simulink model "Sim1"  (R2024b)
settings: Solver=VariableStepAuto  StartTime=0.0  StopTime=50  RelTol=1e-3
undefined symbols (not defined in the file or in its folder): eng, gbx, road, tire, veh
settings Model: Creator=amira  LastModifiedBy=Ali
settings OptimizationCC: ReuseModelBlockBuffer=off
settings RTWCC: GPUComputeCapability=3.5

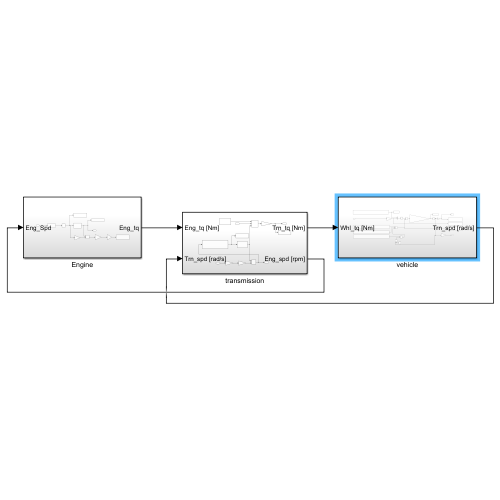
[thumbnail: Simulink's stored preview of the top-level diagram]
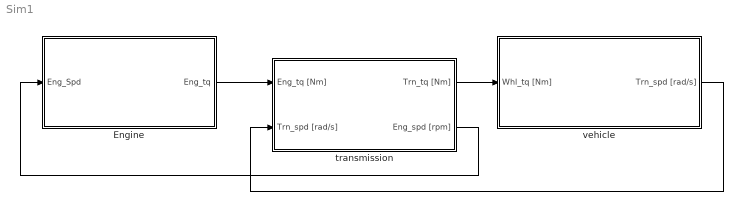
== system Sim1 ==
  Engine : Subsystem
  transmission : Subsystem
  vehicle : Subsystem
  wires:
  Engine/1(Eng_tq) -> transmission/1(Eng_tq [Nm])
  transmission/2(Eng_spd [rpm]) -> Engine/1(Eng_Spd)
  transmission/1(Trn_tq [Nm]) -> vehicle/1(Whl_tq [Nm])
  vehicle/1(Trn_spd [rad/s]) -> transmission/2(Trn_spd [rad/s])

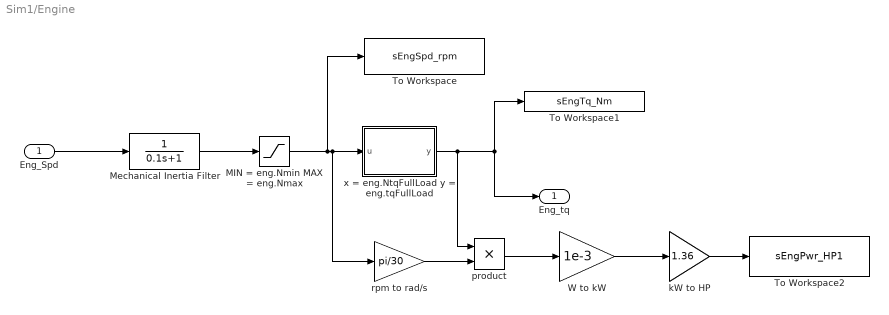
== system Sim1/Engine ==
  Eng_Spd : Inport
  MIN = eng.Nmin MAX = eng.Nmax : Saturate  UpperLimit=6500  LowerLimit=1000
  Mechanical Inertia Filter : TransferFcn  Denominator=[0.1 1]
  To Workspace : ToWorkspace  VariableName=sEngSpd_rpm  SaveFormat=Timeseries  SampleTime=-1
  To Workspace1 : ToWorkspace  VariableName=sEngTq_Nm  SaveFormat=Timeseries  SampleTime=-1
  To Workspace2 : ToWorkspace  VariableName=sEngPwr_HP1  SaveFormat=Timeseries  SampleTime=-1
  W to kW : Gain  Gain=1e-3
  kW to HP : Gain  Gain=1.36
  product : Product
  rpm to rad/s : Gain  Gain=pi/30
  x = eng.NtqFullLoad y = eng.tqFullLoad : MATLAB Function  TreatAsAtomicUnit=on
  Eng_tq : Outport
  wires:
  Eng_Spd/1 -> Mechanical Inertia Filter/1
  Mechanical Inertia Filter/1 -> MIN = eng.Nmin MAX = eng.Nmax/1
  MIN = eng.Nmin MAX = eng.Nmax/1 -> x = eng.NtqFullLoad y = eng.tqFullLoad/1(u), rpm to rad/s/1, To Workspace/1
  x = eng.NtqFullLoad y = eng.tqFullLoad/1(y) -> Eng_tq/1, To Workspace1/1, product/1
  rpm to rad/s/1 -> product/2
  product/1 -> W to kW/1
  W to kW/1 -> kW to HP/1
  kW to HP/1 -> To Workspace2/1

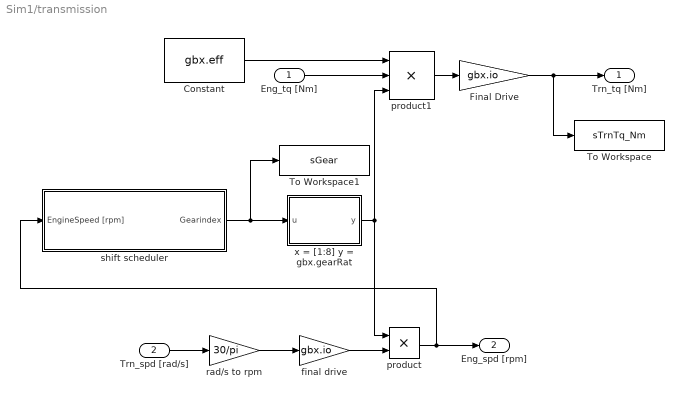
== system Sim1/transmission ==
  Eng_tq [Nm] : Inport
  Trn_spd [rad/s] : Inport  Port=2
  Constant : Constant  Value=gbx.eff
  Final Drive : Gain  Gain=gbx.io
  To Workspace : ToWorkspace  VariableName=sTrnTq_Nm  SaveFormat=Timeseries  SampleTime=-1
  To Workspace1 : ToWorkspace  VariableName=sGear  SaveFormat=Timeseries  SampleTime=-1
  final drive : Gain  Gain=gbx.io
  product : Product
  product1 : Product  Inputs=3
  rad/s to rpm : Gain  Gain=30/pi
  shift scheduler : Subsystem
  x = [1:8] y = gbx.gearRat : MATLAB Function  TreatAsAtomicUnit=on
  Trn_tq [Nm] : Outport
  Eng_spd [rpm] : Outport  Port=2
  wires:
  rad/s to rpm/1 -> final drive/1
  final drive/1 -> product/2
  x = [1:8] y = gbx.gearRat/1(y) -> product/1, product1/3
  Constant/1 -> product1/1
  Eng_tq [Nm]/1 -> product1/2
  product1/1 -> Final Drive/1
  Final Drive/1 -> Trn_tq [Nm]/1, To Workspace/1
  product/1 -> Eng_spd [rpm]/1, shift scheduler/1(EngineSpeed [rpm])
  shift scheduler/1(Gearindex) -> To Workspace1/1, x = [1:8] y = gbx.gearRat/1(u)
  Trn_spd [rad/s]/1 -> rad/s to rpm/1

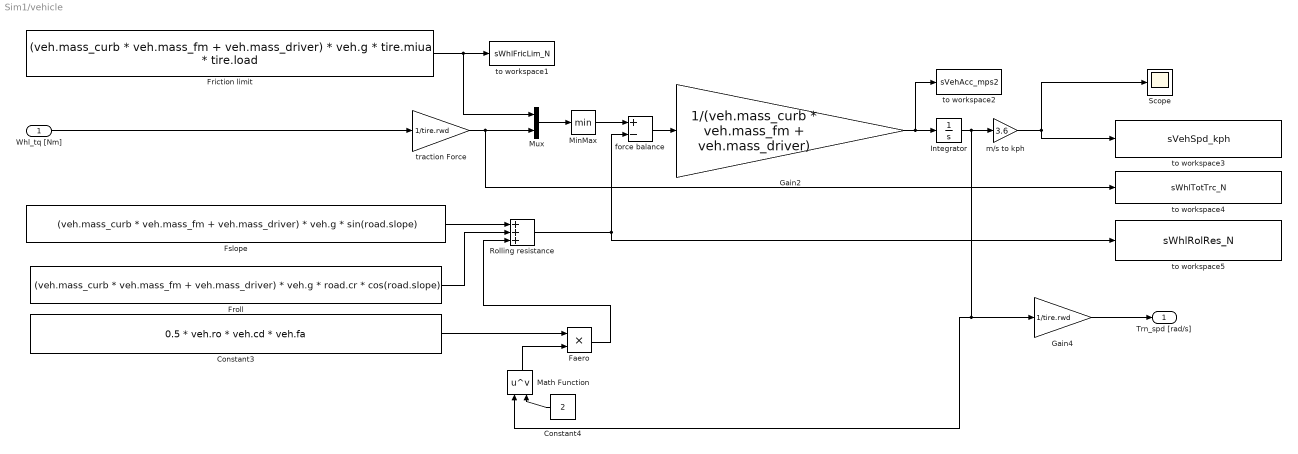
== system Sim1/vehicle ==
  Whl_tq [Nm] : Inport
  Constant3 : Constant  Value=0.5 * veh.ro * veh.cd * veh.fa
  Constant4 : Constant  Value=2
  Faero : Product
  Friction limit : Constant  Value=(veh.mass_curb * veh.mass_fm + veh.mass_driver) * veh.g * tire.miua * tire.load
  Froll : Constant  Value=(veh.mass_curb * veh.mass_fm + veh.mass_driver) * veh.g * road.cr * cos(road.slope)
  Fslope : Constant  Value=(veh.mass_curb * veh.mass_fm + veh.mass_driver) * veh.g * sin(road.slope)
  Gain2 : Gain  Gain=1/(veh.mass_curb * veh.mass_fm + veh.mass_driver)
  Gain4 : Gain  Gain=1/tire.rwd
  Integrator : Integrator
  Math Function : Math  Operator=pow  SignedPower=on
  MinMax : MinMax
  Mux : Mux  Inputs=2
  Rolling resistance : Sum  Inputs=+++
  Scope : Scope
  force balance : Sum  Inputs=+-
  m/s to kph : Gain  Gain=3.6
  to workspace1 : ToWorkspace  VariableName=sWhlFricLim_N  SaveFormat=Timeseries  SampleTime=-1
  to workspace2 : ToWorkspace  VariableName=sVehAcc_mps2  SaveFormat=Timeseries  SampleTime=-1
  to workspace3 : ToWorkspace  VariableName=sVehSpd_kph  SaveFormat=Timeseries  SampleTime=-1
  to workspace4 : ToWorkspace  VariableName=sWhlTotTrc_N  SaveFormat=Timeseries  SampleTime=-1
  to workspace5 : ToWorkspace  VariableName=sWhlRolRes_N  SaveFormat=Timeseries  SampleTime=-1
  traction Force : Gain  Gain=1/tire.rwd
  Trn_spd [rad/s] : Outport
  wires:
  Integrator/1 -> Math Function/1, Gain4/1, m/s to kph/1
  Whl_tq [Nm]/1 -> traction Force/1
  MinMax/1 -> force balance/1
  Gain4/1 -> Trn_spd [rad/s]/1
  Rolling resistance/1 -> force balance/2, to workspace5/1
  Fslope/1 -> Rolling resistance/1
  traction Force/1 -> to workspace4/1, Mux/2
  m/s to kph/1 -> Scope/1, to workspace3/1
  Faero/1 -> Rolling resistance/3
  Froll/1 -> Rolling resistance/2
  Mux/1 -> MinMax/1
  force balance/1 -> Gain2/1
  Constant3/1 -> Faero/1
  Math Function/1 -> Faero/2
  Friction limit/1 -> Mux/1, to workspace1/1
  Constant4/1 -> Math Function/2
  Gain2/1 -> to workspace2/1, Integrator/1

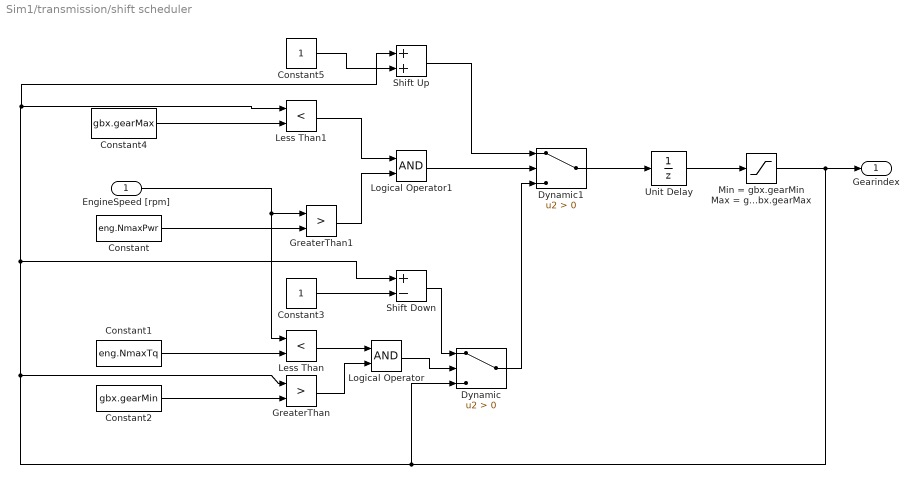
== system Sim1/transmission/shift scheduler ==
  EngineSpeed [rpm] : Inport
  Constant : Constant  Value=eng.NmaxPwr
  Constant1 : Constant  Value=eng.NmaxTq
  Constant2 : Constant  Value=gbx.gearMin
  Constant3 : Constant
  Constant4 : Constant  Value=gbx.gearMax
  Constant5 : Constant
  Dynamic : Switch  Criteria=u2 > Threshold  SaturateOnIntegerOverflow=off  InputSameDT=off
  Dynamic1 : Switch  Criteria=u2 > Threshold  SaturateOnIntegerOverflow=off  InputSameDT=off
  GreaterThan : RelationalOperator  Operator=>  OutDataTypeStr=boolean  RndMeth=Simplest  InputSameDT=off
  GreaterThan1 : RelationalOperator  Operator=>  OutDataTypeStr=boolean  RndMeth=Simplest  InputSameDT=off
  Less Than : RelationalOperator  Operator=<  OutDataTypeStr=boolean  RndMeth=Simplest  InputSameDT=off
  Less Than1 : RelationalOperator  Operator=<  OutDataTypeStr=boolean  RndMeth=Simplest  InputSameDT=off
  Logical Operator : Logic  AllPortsSameDT=off  OutDataTypeStr=boolean
  Logical Operator1 : Logic  AllPortsSameDT=off  OutDataTypeStr=boolean
  Min = gbx.gearMin Max = gbx.gearMax : Saturate  UpperLimit=8  LowerLimit=1
  Shift Down : Sum  Inputs=+-
  Shift Up : Sum
  Unit Delay : UnitDelay  SampleTime=-1  HasFrameUpgradeWarning=on
  Gearindex : Outport
  wires:
  EngineSpeed [rpm]/1 -> Less Than/1, GreaterThan1/1
  Constant1/1 -> Less Than/2
  Constant/1 -> GreaterThan1/2
  Constant2/1 -> GreaterThan/2
  Constant4/1 -> Less Than1/2
  GreaterThan1/1 -> Logical Operator1/2
  Less Than1/1 -> Logical Operator1/1
  Less Than/1 -> Logical Operator/1
  GreaterThan/1 -> Logical Operator/2
  Logical Operator/1 -> Dynamic/2
  Logical Operator1/1 -> Dynamic1/2
  Shift Up/1 -> Dynamic1/1
  Shift Down/1 -> Dynamic/1
  Constant5/1 -> Shift Up/2
  Constant3/1 -> Shift Down/2
  Dynamic/1 -> Dynamic1/3
  Unit Delay/1 -> Min = gbx.gearMin Max = gbx.gearMax/1
  Dynamic1/1 -> Unit Delay/1
  Min = gbx.gearMin Max = gbx.gearMax/1 -> GreaterThan/1, Shift Down/1, Less Than1/1, Shift Up/1, Dynamic/3, Gearindex/1

== matlab function Sim1/Engine/x = eng.NtqFullLoad y = eng.tqFullLoad ==
  data: u input; y output
function y = fcn(u)
Ne= [1000 2020 2990 3500 5000 6500];
Te= [306 385 439 450 450 367];
p = polyfit(Ne,Te,4);
y = p(1)*u^4 + p(2)*u^3 + p(3)*u^2 + p(4)*u + p(5);
end

== matlab function Sim1/transmission/x = [1:8] y = gbx.gearRat ==
  data: u input; y output
function y = fcn(u)
x = [1 2 3 4 5 6 7 8];
gbx.gearRat = [4.71 3.14 2.11 1.67 1.29 1.00 0.84 0.67];
p = polyfit(x,gbx.gearRat,4);
y = p(1)*u^4 + p(2)*u^3 + p(3)*u^2 + p(4)*u + p(5);
end
